simulink model "Variable_Frequency_Sine_Wave12"  (R2020a)
settings: Solver=VariableStepAuto  StartTime=0.0  StopTime=1  RelTol=1e-3
settings Model: Creator=hp  LastModifiedBy=hp

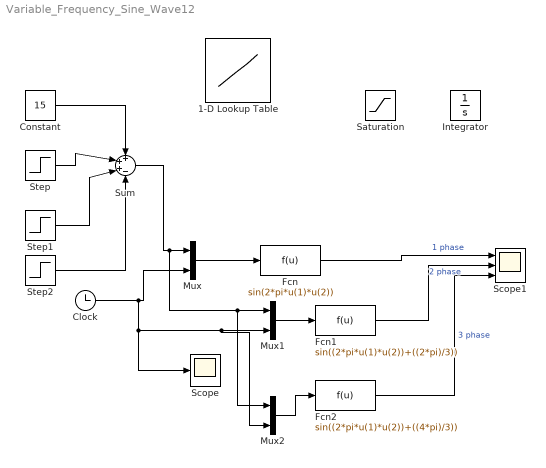
== system Variable_Frequency_Sine_Wave12 ==
  1-D Lookup Table : Lookup_n-D  NumberOfTableDimensions=1  BreakpointsSpecification=Even spacing  BreakpointsForDimension1=[0:5]  BreakpointsForDimension1FirstPoint=3000  BreakpointsForDimension1Spacing=50  BreakpointsForDimension1Min=0  BreakpointsForDimension1Max=50  Table=[15:50]  InternalRulePriority=Speed  RndMeth=Simplest  InputSameDT=on
  Clock : Clock
  Constant : Constant  Value=15
  Fcn : Fcn  Expr=sin(2*pi*u(1)*u(2))
  Fcn1 : Fcn  Expr=sin((2*pi*u(1)*u(2))+((2*pi)/3))
  Fcn2 : Fcn  Expr=sin((2*pi*u(1)*u(2))+((4*pi)/3))
  Integrator : Integrator
  Mux : Mux  Inputs=2
  Mux1 : Mux  Inputs=2
  Mux2 : Mux  Inputs=2
  Saturation : Saturate  UpperLimit=50  LowerLimit=0
  Scope : Scope
  Scope1 : Scope  NumInputPorts=3
  Step : Step  Time=.2  After=15  SampleTime=1e-6
  Step1 : Step  Time=.4  After=20  SampleTime=1e-6
  Step2 : Step  Time=.6  After=40  SampleTime=1e-6
  Sum : Sum  Inputs=+++-
  wires:
  Clock/1 -> Mux2/2, Mux1/2, Scope/1, Mux/2
  Step/1 -> Sum/2
  Constant/1 -> Sum/1
  Step1/1 -> Sum/3
  Sum/1 -> Mux2/1, Mux1/1, Mux/1
  Mux/1 -> Fcn/1
  Fcn/1 -> Scope1/1  "1 phase"
  Step2/1 -> Sum/4
  Mux1/1 -> Fcn1/1
  Mux2/1 -> Fcn2/1
  Fcn1/1 -> Scope1/2  "2 phase"
  Fcn2/1 -> Scope1/3  "3 phase"
